simulink library "rotorTorqueCtrlFeedBackLinearized"  (R2022a)
settings: Solver=VariableStepAuto  StartTime=0.0  StopTime=10.0  RelTol=1e-3
undefined symbols (not defined in the file): rho, vhcl
libraries: sixDoFDynamicsCoupledFossenTurbDynamics x1, localApparentWind_ul x1
settings Model: Creator=adabney  LastModifiedBy=adabney

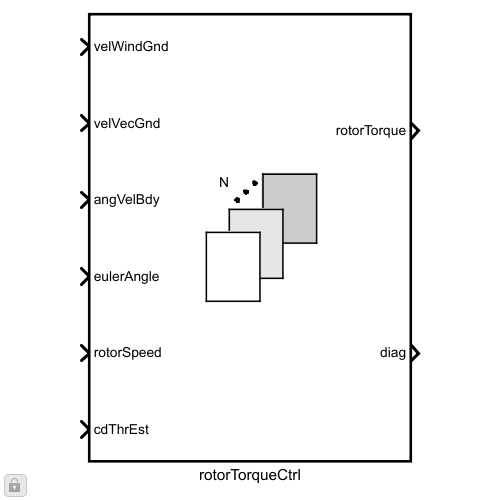
[thumbnail: Simulink's stored preview of the top-level diagram]
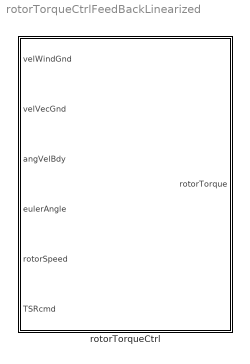
== system rotorTorqueCtrlFeedBackLinearized ==
  rotorTorqueCtrl : Subsystem  TreatAsAtomicUnit=on  mask{turb_struct=vhcl.struct('OCT.turb'), rho=rho}
      mask prompts: turb_struct "Turbine Structures"; rho "Fluid Density"

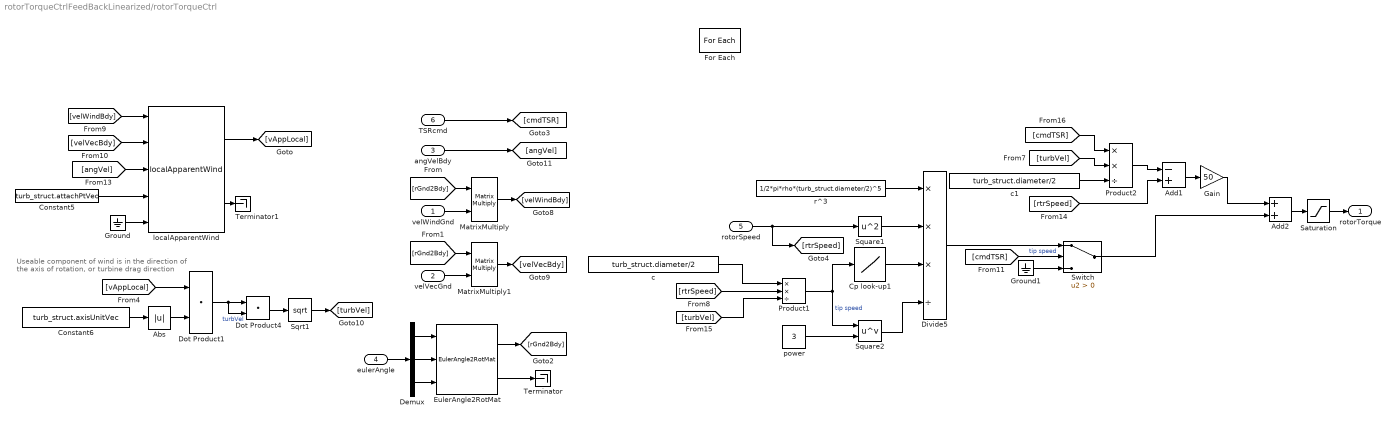
== system rotorTorqueCtrlFeedBackLinearized/rotorTorqueCtrl ==
  note: Useable component of wind is in the direction of
      | the axis of rotation, or turbine drag direction
  velWindGnd : Inport
  velVecGnd : Inport  Port=2
  angVelBdy : Inport  Port=3
  eulerAngle : Inport  Port=4
  rotorSpeed : Inport  Port=5  Partition=on  PartitionDimension=1  PartitionWidth=1  PartitionOffset=0
  TSRcmd : Inport  Port=6
  Abs : Abs  SaturateOnIntegerOverflow=off
  Add1 : Sum  Inputs=-+
  Add2 : Sum
  Constant5 : Constant  Value=turb_struct.attachPtVec
  Constant6 : Constant  Value=turb_struct.axisUnitVec
  Cp look-up1 : Lookup_n-D  NumberOfTableDimensions=1  BreakpointsForDimension1=turb_struct.RPMref  Table=turb_struct.CpLookup  InternalRulePriority=Speed  RndMeth=Simplest
  Demux : Demux  Outputs=3
  Divide5 : Product  Inputs=***/
  Dot Product1 : DotProduct  OutDataTypeStr=Inherit: Inherit via internal rule
  Dot Product4 : DotProduct  OutDataTypeStr=Inherit: Inherit via internal rule
  EulerAngle2RotMat : sixDoFDynamicsCoupledFossenTurbDynamics/sixDoFDynamicsCoupledFossenTurbDynamics/EulerAngle2RotMat  SystemSampleTime=-1  VariantActivationTime=update diagram  Latency=0  AutoFrameSizeCalculation=off
  For Each : ForEach  DisableCoverage=on  IterateSubsysMaskParameter=on,off  SubsysMaskParameterIterationDimension=2,1  SubsysMaskParameterIterationStepSize=1,1
  Gain : Gain  Gain=50
  Ground : Ground
  Ground1 : Ground
  MatrixMultiply : Product  Multiplication=Matrix(*)
  MatrixMultiply1 : Product  Multiplication=Matrix(*)
  Product1 : Product  Inputs=**/
  Product2 : Product  Inputs=**/
  Saturation : Saturate  UpperLimit=turb_struct.torqueLim  LowerLimit=-turb_struct.torqueLim
  Sqrt1 : Sqrt
  Square1 : Math  Operator=square
  Square2 : Math  Operator=pow
  Switch : Switch  Criteria=u2 > Threshold  SaturateOnIntegerOverflow=off  InputSameDT=off
  Terminator : Terminator
  Terminator1 : Terminator
  c : Constant  Value=turb_struct.diameter/2
  c1 : Constant  Value=turb_struct.diameter/2
  localApparentWind : localApparentWind_ul/localApparentWind  SystemSampleTime=-1  VariantActivationTime=update diagram  Latency=0  AutoFrameSizeCalculation=off
  power : Constant  Value=3
  r^3 : Constant  Value=1/2*pi*rho*(turb_struct.diameter/2)^5
  rotorTorque : Outport  ConcatenationDimension=1
  wires:
  [vAppLocal] -> Dot Product1/1
  Constant6/1 -> Abs/1
  Abs/1 -> Dot Product1/2
  Dot Product4/1 -> Sqrt1/1
  Dot Product1/1 -> Dot Product4/1, Dot Product4/2  "turbVel"
  Ground/1 -> localApparentWind/5
  Constant5/1 -> localApparentWind/4
  localApparentWind/1 -> [vAppLocal]
  localApparentWind/2 -> Terminator1/1
  [angVel] -> localApparentWind/3
  EulerAngle2RotMat/1 -> [rGnd2Bdy]
  Demux/3 -> EulerAngle2RotMat/3
  Demux/1 -> EulerAngle2RotMat/1
  EulerAngle2RotMat/2 -> Terminator/1
  eulerAngle/1 -> Demux/1
  Demux/2 -> EulerAngle2RotMat/2
  [velWindBdy] -> localApparentWind/1
  [velVecBdy] -> localApparentWind/2
  power/1 -> Square2/2
  Cp look-up1/1 -> Divide5/3
  Square1/1 -> Divide5/2
  Square2/1 -> Divide5/4
  r^3/1 -> Divide5/1
  Product1/1 -> Cp look-up1/1, Square2/1  "tip speed"
  rotorSpeed/1 -> [rtrSpeed], Square1/1
  [rGnd2Bdy] -> MatrixMultiply1/1
  [rGnd2Bdy] -> MatrixMultiply/1
  velVecGnd/1 -> MatrixMultiply1/2
  velWindGnd/1 -> MatrixMultiply/2
  MatrixMultiply/1 -> [velWindBdy]
  MatrixMultiply1/1 -> [velVecBdy]
  angVelBdy/1 -> [angVel]
  Divide5/1 -> Switch/1
  Saturation/1 -> rotorTorque/1
  Ground1/1 -> Switch/3
  Switch/1 -> Add2/2
  [cmdTSR] -> Switch/2  "tip speed"
  TSRcmd/1 -> [cmdTSR]
  c/1 -> Product1/1
  [rtrSpeed] -> Product1/2
  [turbVel] -> Product2/2
  c1/1 -> Product2/3
  Product2/1 -> Add1/1
  [rtrSpeed] -> Add1/2
  Add1/1 -> Gain/1
  Add2/1 -> Saturation/1
  Sqrt1/1 -> [turbVel]
  [turbVel] -> Product1/3
  Gain/1 -> Add2/1
  [cmdTSR] -> Product2/1
